simulink model "neural_controller"  (R2017a)
settings: Solver=FixedStepDiscrete  StartTime=0.0  StopTime=inf  FixedStep=0.002  RelTol=1e-3  EnableMultiTasking=on
undefined symbols (not defined in the file or in its folder): HIL
libraries: neural x136, quarc_library x4, simulink x1
(part 3 of 4)

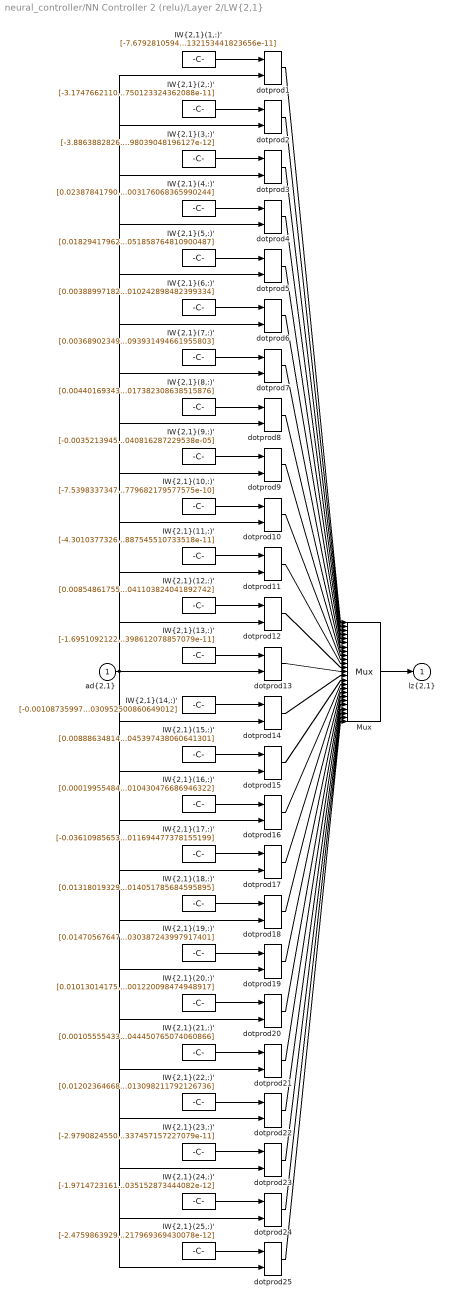
== system neural_controller/NN Controller 2 (relu)/Layer 2/LW{2,1} ==
  "ad{2,1}" : Inport  PortDimensions=25
      mask Display: e = 0.06;c1 = [120 230 180]/255;c2 = ([120 230 180]+0)/(256+128);c3 = ([120 230 180]+128)/(256+128);patch([0 1 1 0],[0 0 1 1],c1);patch([0 1 1 1-e 1-e 0+e],[0 0 1 1-e 0+e 0+e],c2);patch([0 0 1 1-e 0+e 0+e],[0 1 1 1-e 1-e 0+e],c3);plot([0 1 1 0 0],[0 0 1 1 0]);
  "IW{2,1}(1,:)'" : Constant  Value=[-7.6792810594584661e-09;-7.1126316738020698e-11;1.7998320918344641e-08;-2.003723626458679e-10;-1.8516180965883707e-10;-7.5860076472246306e-11;6.2299829523009267e-10;-1.0515209795277028e-10;-1.8827427881449038e-09;2.218470791657716e-11;-3.9406915599531058e-08;1.0151503705757366e-12;-1.9023546382725779e-08;-2.2032313786793295e-10;-2.3151757914767001e-09;-2.9984532169035445e-11;-9.5093536671353531e-12;-5.0992263322406924e-08;-1.3344982605011259e-08;-2.9158255260832613e-09;-1.1630319166261373e-10;-1.2964229482817726e-08;6.1084505465677229e-09;1.0825281524140743e-10;1.8132153441823656e-11]
      mask Display: e = 0.06;c1 = [120 150 230]/255;c2 = ([120 150 230]+0)/383;c3 = ([120 150 230]+128)/383;patch([0 1 1 0],[0 0 1 1],c1);patch([0 1 1 1-e 1-e 0+e],[0 0 1 1-e 0+e 0+e],c2);patch([0 0 1 1-e 0+e 0+e],[0 1 1 1-e 1-e 0+e],c3);plot([0 1 1 0 0],[0 0 1 1 0]);disp('weights');
  "IW{2,1}(10,:)'" : Constant  Value=[-7.539833734705316e-11;-2.4411431451428775e-10;5.9162341033399517e-11;-5.48070123741515e-10;-4.5302392434479749e-10;-2.5669878462677975e-10;1.7387695818048645e-10;-2.2463697075379773e-10;-1.5814520153849316e-10;-1.6547463732050574e-10;-2.9538417906818055e-10;-3.7654524057014066e-12;-2.5148569538890934e-10;-5.7656949292448e-10;2.5000753899474519e-12;-2.4840785547122653e-10;6.2010400842961357e-11;-1.630706221709544e-10;-2.1704856737930736e-10;-8.2373025243356772e-11;-2.9314899085759011e-10;1.8311770093531284e-10;-2.5372084254757587e-10;-4.0386388939167889e-11;-1.2779682179577575e-10]
      mask Display: e = 0.06;c1 = [120 150 230]/255;c2 = ([120 150 230]+0)/383;c3 = ([120 150 230]+128)/383;patch([0 1 1 0],[0 0 1 1],c1);patch([0 1 1 1-e 1-e 0+e],[0 0 1 1-e 0+e 0+e],c2);patch([0 0 1 1-e 0+e 0+e],[0 1 1 1-e 1-e 0+e],c3);plot([0 1 1 0 0],[0 0 1 1 0]);disp('weights');
  "IW{2,1}(11,:)'" : Constant  Value=[-4.301037732631331e-11;-2.569410134808951e-12;-1.0469632599092887e-11;-1.2595773712822758e-12;-1.0156678735682078e-11;-3.4054838340213689e-11;-9.5770075392691075e-12;-1.8306926198411783e-12;-1.0308441497359357e-10;-9.5984236805500613e-11;-1.8259977268230217e-10;-1.9587259074091726e-11;-1.3968105946278729e-10;-1.1647665091168313e-11;-1.3851019848052193e-11;-9.6033937176644037e-12;2.820579720713071e-11;-1.0067866005581733e-10;-1.3484847526334624e-10;-5.6651723409524551e-11;8.5942338897835642e-12;-4.1233821262441008e-12;-1.1667206126410447e-10;-2.6214250577623542e-12;-6.6887545510733518e-11]
      mask Display: e = 0.06;c1 = [120 150 230]/255;c2 = ([120 150 230]+0)/383;c3 = ([120 150 230]+128)/383;patch([0 1 1 0],[0 0 1 1],c1);patch([0 1 1 1-e 1-e 0+e],[0 0 1 1-e 0+e 0+e],c2);patch([0 0 1 1-e 0+e 0+e],[0 1 1 1-e 1-e 0+e],c3);plot([0 1 1 0 0],[0 0 1 1 0]);disp('weights');
  "IW{2,1}(12,:)'" : Constant  Value=[0.0085486175547883157;0.038921469431951253;0.00072928454322535984;-0.005919310881027433;0.0067324029361368288;0.0014729867062613932;0.011651872976152538;0.0096951132432792075;0.014282980967113987;-0.0022472072990480309;0.02697281453022778;0.0033402977445982814;0.066526733165617802;0.0027361323723594641;0.0009416351130375817;0.0060005892677358922;-0.0017547579068491084;0.011895645295689969;0.0058107012873306555;-0.005567481289830826;0.10457499147972557;0.011928304424710184;0.0010842351755472252;0.03450444048361162;0.0041103824041892742]
      mask Display: e = 0.06;c1 = [120 150 230]/255;c2 = ([120 150 230]+0)/383;c3 = ([120 150 230]+128)/383;patch([0 1 1 0],[0 0 1 1],c1);patch([0 1 1 1-e 1-e 0+e],[0 0 1 1-e 0+e 0+e],c2);patch([0 0 1 1-e 0+e 0+e],[0 1 1 1-e 1-e 0+e],c3);plot([0 1 1 0 0],[0 0 1 1 0]);disp('weights');
  "IW{2,1}(13,:)'" : Constant  Value=[-1.6951092122585871e-08;-5.9712221408849155e-11;-4.2727995881829927e-08;-1.5268723788522534e-10;-1.1786285260925152e-10;-6.1318022475459716e-11;-1.4492083639181336e-09;-7.120193341696578e-11;-5.8746453350967224e-09;-1.522926600548734e-11;-7.6277173675718993e-08;5.0409460013806238e-13;-3.5200837251621827e-08;-1.6739184538221271e-10;-5.201417827921483e-09;-7.5605015966112313e-11;7.8486292035284465e-12;-1.0740901393181189e-07;-2.130777853307425e-08;-1.0927906376289981e-09;-7.458065697127481e-11;-5.1051051799692016e-08;-1.3959719228474327e-08;-1.2266524690474954e-11;-1.1398612078857079e-11]
      mask Display: e = 0.06;c1 = [120 150 230]/255;c2 = ([120 150 230]+0)/383;c3 = ([120 150 230]+128)/383;patch([0 1 1 0],[0 0 1 1],c1);patch([0 1 1 1-e 1-e 0+e],[0 0 1 1-e 0+e 0+e],c2);patch([0 0 1 1-e 0+e 0+e],[0 1 1 1-e 1-e 0+e],c3);plot([0 1 1 0 0],[0 0 1 1 0]);disp('weights');
  "IW{2,1}(14,:)'" : Constant  Value=[-0.001087359976365982;0.014994532054224833;-0.00048161962687797658;0.0023381707521366577;0.034947327362041904;0.010589180365643583;0.00037580858668208783;0.0044711535329865354;0.0051232386073423886;-0.00024523223986675933;-0.020647122052367812;0.0037805115068640094;0.12739374876765761;0.030452209012630911;-0.00087797584990192935;0.015370265125823646;-0.038906996003827653;-0.027759582662904993;-0.0086574652701497598;0.013807193556461107;0.062866770256710017;0.008848576139869082;7.7852200123227166e-05;0.066823430685743548;0.0030952500860649012]
      mask Display: e = 0.06;c1 = [120 150 230]/255;c2 = ([120 150 230]+0)/383;c3 = ([120 150 230]+128)/383;patch([0 1 1 0],[0 0 1 1],c1);patch([0 1 1 1-e 1-e 0+e],[0 0 1 1-e 0+e 0+e],c2);patch([0 0 1 1-e 0+e 0+e],[0 1 1 1-e 1-e 0+e],c3);plot([0 1 1 0 0],[0 0 1 1 0]);disp('weights');
  "IW{2,1}(15,:)'" : Constant  Value=[0.0088863481441649201;0.028805562177555567;0.00085740479293599928;-0.010448278624971764;-0.014559925730524618;-0.0052039232464403118;0.010078670622544418;0.0069288194214313942;0.012410948017324149;5.9244647332985789e-05;0.036181882849986205;0.0014764956348752136;0.01593110490784052;-0.017219733564965121;0.001196341715713193;-0.002033634151277173;0.010431016127799078;0.022044008297568363;0.0076614564960669745;-0.018076495184618409;0.0729467409982682;0.010576460114962811;0.0010004496153833981;-0.0063583331762361835;0.0045397438060641301]
      mask Display: e = 0.06;c1 = [120 150 230]/255;c2 = ([120 150 230]+0)/383;c3 = ([120 150 230]+128)/383;patch([0 1 1 0],[0 0 1 1],c1);patch([0 1 1 1-e 1-e 0+e],[0 0 1 1-e 0+e 0+e],c2);patch([0 0 1 1-e 0+e 0+e],[0 1 1 1-e 1-e 0+e],c3);plot([0 1 1 0 0],[0 0 1 1 0]);disp('weights');
  "IW{2,1}(16,:)'" : Constant  Value=[0.00019955484401158415;0.00067388635728634315;1.8997775731461967e-05;-0.0002256414614354404;-0.00027635177889485691;-0.00010088774089898898;0.00023091529890104565;0.00016289364059207442;0.0002845954187697474;1.1933203969252801e-05;0.00079394575255332988;3.7722143976141233e-05;0.00055021284806064342;-0.0003394896127411838;2.6308884670988423e-05;-2.6041962717278154e-05;0.00020427353166977094;0.0004715896170833154;0.00016821614579598878;-0.00037881141697235915;0.0017132367012811396;0.000250579116094033;2.2688109769553548e-05;-5.2576931568082683e-05;0.00010430476686946322]
      mask Display: e = 0.06;c1 = [120 150 230]/255;c2 = ([120 150 230]+0)/383;c3 = ([120 150 230]+128)/383;patch([0 1 1 0],[0 0 1 1],c1);patch([0 1 1 1-e 1-e 0+e],[0 0 1 1-e 0+e 0+e],c2);patch([0 0 1 1-e 0+e 0+e],[0 1 1 1-e 1-e 0+e],c3);plot([0 1 1 0 0],[0 0 1 1 0]);disp('weights');
  "IW{2,1}(17,:)'" : Constant  Value=[-0.036109856536489467;-0.019036186629064276;-0.0054815016316539381;0.06967861303102571;0.061332727846017877;0.0052795114685041198;-0.0051925191815313833;-0.0018808362547497175;-0.0051001745228906395;-0.98650212883476152;-0.29053726241657934;-0.01599267235973249;1.2449192312731583;0.027313731780371622;-0.0091790878449782738;0.0098279050215846452;-0.27375674339103112;-0.27079956763634183;-0.059001072253794591;0.14671588527890911;0.24543718884772109;0.041228611003460536;-0.002497278540755815;1.0645004239809719;-0.00011694477378155199]
      mask Display: e = 0.06;c1 = [120 150 230]/255;c2 = ([120 150 230]+0)/383;c3 = ([120 150 230]+128)/383;patch([0 1 1 0],[0 0 1 1],c1);patch([0 1 1 1-e 1-e 0+e],[0 0 1 1-e 0+e 0+e],c2);patch([0 0 1 1-e 0+e 0+e],[0 1 1 1-e 1-e 0+e],c3);plot([0 1 1 0 0],[0 0 1 1 0]);disp('weights');
  "IW{2,1}(18,:)'" : Constant  Value=[0.013180193294562671;-0.01832335242095794;0.0018687300632919601;-0.026598429671250812;-0.1192523831811606;-0.037681292647196066;0.0046595445016668511;-0.0062180779326500889;0.0050876623668604619;0.0027113534960816889;0.094353915225575083;-0.008205881294492191;-0.29794094749763644;-0.11288884666587964;0.0030523700333772424;-0.043573015575918687;0.083582031303561524;0.085431764893414724;0.020105502131936188;-0.07162657266632845;-0.049990786533464941;-0.0061687796055690811;0.00099094026683705337;-0.21300169631618429;0.0014051785684595895]
      mask Display: e = 0.06;c1 = [120 150 230]/255;c2 = ([120 150 230]+0)/383;c3 = ([120 150 230]+128)/383;patch([0 1 1 0],[0 0 1 1],c1);patch([0 1 1 1-e 1-e 0+e],[0 0 1 1-e 0+e 0+e],c2);patch([0 0 1 1-e 0+e 0+e],[0 1 1 1-e 1-e 0+e],c3);plot([0 1 1 0 0],[0 0 1 1 0]);disp('weights');
  "IW{2,1}(19,:)'" : Constant  Value=[0.014705676471526079;-0.0037914905499059136;0.0019320217527694461;-0.025167320520140802;-0.10492667645076631;-0.033242947282169116;0.0080510037261118644;-0.0024456617849274625;0.0092923766451942381;0.0064911713473241785;0.093334108146343672;-0.006350500228105049;-0.24268427749482493;-0.10005757905756707;0.0030711877779970023;-0.03757539071369137;0.0750431051703635;0.080824464711242633;0.02014862419218081;-0.065499627476395386;-0.01266812952475955;-0.0030906270795722146;0.0012441033357813963;-0.18256389585322375;0.0030387243997917401]
      mask Display: e = 0.06;c1 = [120 150 230]/255;c2 = ([120 150 230]+0)/383;c3 = ([120 150 230]+128)/383;patch([0 1 1 0],[0 0 1 1],c1);patch([0 1 1 1-e 1-e 0+e],[0 0 1 1-e 0+e 0+e],c2);patch([0 0 1 1-e 0+e 0+e],[0 1 1 1-e 1-e 0+e],c3);plot([0 1 1 0 0],[0 0 1 1 0]);disp('weights');
  "IW{2,1}(2,:)'" : Constant  Value=[-3.1747662110966132e-11;7.73937278117594e-12;-3.7463219540287004e-12;-5.9340728255523212e-12;-2.7236647618137786e-12;-4.1883456193740931e-11;7.3694992314728212e-12;-5.3344196383348506e-12;-8.7351651384151508e-11;-7.9982925418328494e-11;-1.4012840818143832e-10;2.8438846222131151e-13;-1.2681316049939503e-10;7.3261463691447547e-13;5.4642931551664244e-12;-1.089076241700762e-11;2.7946339069716205e-11;-9.3284990243965443e-11;-1.11098224269136e-10;-3.736233021564739e-11;-7.9185065671258803e-12;-3.0588242026652366e-12;-8.9017375531224679e-11;-6.9971911726714913e-12;-5.9750123324362088e-11]
      mask Display: e = 0.06;c1 = [120 150 230]/255;c2 = ([120 150 230]+0)/383;c3 = ([120 150 230]+128)/383;patch([0 1 1 0],[0 0 1 1],c1);patch([0 1 1 1-e 1-e 0+e],[0 0 1 1-e 0+e 0+e],c2);patch([0 0 1 1-e 0+e 0+e],[0 1 1 1-e 1-e 0+e],c3);plot([0 1 1 0 0],[0 0 1 1 0]);disp('weights');
  "IW{2,1}(20,:)'" : Constant  Value=[0.01013014175968649;-0.012498606566109946;0.0014217919376139812;-0.020054657772299561;-0.089034158417902326;-0.028145101298815103;0.0038530043220075688;-0.0043517726616277711;0.0042539109661922422;0.0023176727735163783;0.07138270917046452;-0.0060402592245098457;-0.22057473042871267;-0.084368781405189761;0.0023142735131922764;-0.032444695474066011;0.062510062082378234;0.064283472519066437;0.015236329799494694;-0.053744888778392952;-0.034332235462831671;-0.004380518498234549;0.00077480771766379175;-0.15847776405368666;0.001220098474948917]
      mask Display: e = 0.06;c1 = [120 150 230]/255;c2 = ([120 150 230]+0)/383;c3 = ([120 150 230]+128)/383;patch([0 1 1 0],[0 0 1 1],c1);patch([0 1 1 1-e 1-e 0+e],[0 0 1 1-e 0+e 0+e],c2);patch([0 0 1 1-e 0+e 0+e],[0 1 1 1-e 1-e 0+e],c3);plot([0 1 1 0 0],[0 0 1 1 0]);disp('weights');
  "IW{2,1}(21,:)'" : Constant  Value=[0.0010555543300518626;0.0023108869952085005;0.0001140340737172354;-0.00025764674535415014;-0.0020335206928141164;-0.00058363194677767572;0.001015976733930024;0.00052194830220383156;0.0012309537990337566;0.003034245357927848;0.0048571066358807837;-1.8010474050515614e-05;-0.0008171736385963733;-0.0017489116216457131;0.00016742115958282228;-0.00087395919779840981;0.0025258608252747075;0.003543992638676247;0.001082027204315366;-0.001097462565089292;0.0058817508995198005;0.00034873951397666178;0.00011061896876775222;-0.0044380792174932128;0.00044450765074060866]
      mask Display: e = 0.06;c1 = [120 150 230]/255;c2 = ([120 150 230]+0)/383;c3 = ([120 150 230]+128)/383;patch([0 1 1 0],[0 0 1 1],c1);patch([0 1 1 1-e 1-e 0+e],[0 0 1 1-e 0+e 0+e],c2);patch([0 0 1 1-e 0+e 0+e],[0 1 1 1-e 1-e 0+e],c3);plot([0 1 1 0 0],[0 0 1 1 0]);disp('weights');
  "IW{2,1}(22,:)'" : Constant  Value=[0.012023646685503486;-0.016399430115259794;0.0017018603737024665;-0.024187042019239234;-0.10826527256253048;-0.034212024819136842;0.0043048788639688433;-0.0055871994122124952;0.0047097629344176519;0.0025198123677603848;0.08584774552995264;-0.0074326278451825583;-0.27011784762739205;-0.1025051592933013;0.0027781963276783334;-0.039541089455444045;0.075902692834493829;0.077660275130396486;0.01829807684096452;-0.065080988432472217;-0.044788325508654553;-0.0055555191917417736;0.00090661600083301471;-0.19326722570943877;0.0013098211792126736]
      mask Display: e = 0.06;c1 = [120 150 230]/255;c2 = ([120 150 230]+0)/383;c3 = ([120 150 230]+128)/383;patch([0 1 1 0],[0 0 1 1],c1);patch([0 1 1 1-e 1-e 0+e],[0 0 1 1-e 0+e 0+e],c2);patch([0 0 1 1-e 0+e 0+e],[0 1 1 1-e 1-e 0+e],c3);plot([0 1 1 0 0],[0 0 1 1 0]);disp('weights');
  "IW{2,1}(23,:)'" : Constant  Value=[-2.9790824550855467e-11;-6.7120041648906037e-12;-6.0710388600701187e-12;6.8111926946723483e-12;-5.5918771044053318e-12;-5.3716588982021376e-11;7.9204399064392267e-12;-5.5304411013147432e-12;-7.5039652324621861e-11;-1.0979642221447759e-10;-1.8111541917972868e-10;3.6036422567674355e-12;-1.5013353143239249e-10;9.0631795082439541e-12;5.2001717775712573e-12;-8.8846756284766574e-12;5.63369993660505e-11;-8.5663089865284052e-11;-1.4975922319933572e-10;-5.9087910834320275e-11;-1.0976094864108302e-11;-2.2821567234195566e-13;-1.4970013468618046e-10;-3.3131798289421769e-12;-6.2337457157227079e-11]
      mask Display: e = 0.06;c1 = [120 150 230]/255;c2 = ([120 150 230]+0)/383;c3 = ([120 150 230]+128)/383;patch([0 1 1 0],[0 0 1 1],c1);patch([0 1 1 1-e 1-e 0+e],[0 0 1 1-e 0+e 0+e],c2);patch([0 0 1 1-e 0+e 0+e],[0 1 1 1-e 1-e 0+e],c3);plot([0 1 1 0 0],[0 0 1 1 0]);disp('weights');
  "IW{2,1}(24,:)'" : Constant  Value=[-1.9714723161235487e-08;-1.3311802408656901e-11;-4.9745597367239057e-08;-6.1238141909267851e-11;-4.2614013203396124e-11;-2.3751047097339415e-11;-1.745875273838354e-09;-3.1262103553802386e-11;-6.8354121169121968e-09;8.7310823753937401e-12;-8.8780927138340762e-08;8.0689172792817247e-12;-4.0962718389567205e-08;-6.2470140106632016e-11;-6.0661601179792033e-09;-2.5213412563616569e-11;7.8936008881057203e-12;-1.2503704972089463e-07;-2.4798288765834444e-08;-1.2716629166235479e-09;-2.9027139286619137e-11;-5.9460050217482082e-08;-1.62340634639263e-08;-4.9024978961031713e-12;-7.0035152873444082e-12]
      mask Display: e = 0.06;c1 = [120 150 230]/255;c2 = ([120 150 230]+0)/383;c3 = ([120 150 230]+128)/383;patch([0 1 1 0],[0 0 1 1],c1);patch([0 1 1 1-e 1-e 0+e],[0 0 1 1-e 0+e 0+e],c2);patch([0 0 1 1-e 0+e 0+e],[0 1 1 1-e 1-e 0+e],c3);plot([0 1 1 0 0],[0 0 1 1 0]);disp('weights');
  "IW{2,1}(25,:)'" : Constant  Value=[-2.475986392916212e-13;3.5103342751277571e-12;-9.8865432036178798e-13;-3.5781105996286831e-12;1.680453648264645e-12;-9.6435387752281322e-12;1.0839671257044466e-11;-2.3333112413265369e-12;1.6145227362107734e-12;1.0115844357104876e-11;-1.538545584278366e-12;2.9877405143791139e-12;-2.8217741190457491e-12;-3.9461352801403112e-12;-4.4909212344171345e-12;-7.9977565770615599e-12;-1.060594336853036e-11;4.0170778869260341e-12;-1.1289924220125142e-11;-4.8803933824043864e-12;-5.6637584597085797e-12;-1.1211366451726339e-11;-9.5086920530415099e-12;-1.151744751485061e-11;3.7217969369430078e-12]
      mask Display: e = 0.06;c1 = [120 150 230]/255;c2 = ([120 150 230]+0)/383;c3 = ([120 150 230]+128)/383;patch([0 1 1 0],[0 0 1 1],c1);patch([0 1 1 1-e 1-e 0+e],[0 0 1 1-e 0+e 0+e],c2);patch([0 0 1 1-e 0+e 0+e],[0 1 1 1-e 1-e 0+e],c3);plot([0 1 1 0 0],[0 0 1 1 0]);disp('weights');
  "IW{2,1}(3,:)'" : Constant  Value=[-3.8863882826729515e-09;-8.7236645198992326e-12;3.603970721654519e-08;-1.3068868183421996e-12;-8.8122735546962376e-12;-4.6246450436710954e-13;1.0991473834563901e-09;-1.2758449091279944e-11;-4.0923785625092889e-10;9.9829927787223455e-12;-2.3343407056799743e-08;-1.0901018109940021e-11;-1.1834518554835639e-08;-1.3831962085446307e-11;-1.1263358741748662e-09;-2.6282185273417534e-12;6.030387567680668e-12;-2.7312714252359086e-08;-9.4073995884136889e-09;-3.2171861696791232e-09;2.3823661788556188e-12;6.879364424677771e-10;1.205865400955216e-08;1.514331898645933e-11;-9.98039048196127e-12]
      mask Display: e = 0.06;c1 = [120 150 230]/255;c2 = ([120 150 230]+0)/383;c3 = ([120 150 230]+128)/383;patch([0 1 1 0],[0 0 1 1],c1);patch([0 1 1 1-e 1-e 0+e],[0 0 1 1-e 0+e 0+e],c2);patch([0 0 1 1-e 0+e 0+e],[0 1 1 1-e 1-e 0+e],c3);plot([0 1 1 0 0],[0 0 1 1 0]);disp('weights');
  "IW{2,1}(4,:)'" : Constant  Value=[0.023878417904000863;-0.026067123922636486;0.0033203552658731613;-0.046287947654255666;-0.20405883993665144;-0.064518773346212935;0.0096642450015254171;-0.0093423842999586643;0.010764473783257986;0.0063257525323914621;0.16582613371364668;-0.013666627067893646;-0.50147756431859714;-0.19349335838728962;0.0053871303198584474;-0.07422422969371667;0.14364050361718231;0.14857415439413277;0.035450735080039021;-0.12364579065246271;-0.072101489894464063;-0.0095528834486976241;0.0018545884474377983;-0.36234904272976431;0.003176068365990244]
      mask Display: e = 0.06;c1 = [120 150 230]/255;c2 = ([120 150 230]+0)/383;c3 = ([120 150 230]+128)/383;patch([0 1 1 0],[0 0 1 1],c1);patch([0 1 1 1-e 1-e 0+e],[0 0 1 1-e 0+e 0+e],c2);patch([0 0 1 1-e 0+e 0+e],[0 1 1 1-e 1-e 0+e],c3);plot([0 1 1 0 0],[0 0 1 1 0]);disp('weights');
  "IW{2,1}(5,:)'" : Constant  Value=[0.018294179623996869;0.011227153801094326;0.0022556724162024954;-0.025946401053448691;-0.10220234080882376;-0.032391284905276416;0.01273968934703386;0.0012595522230328963;0.015026381503079058;0.013881688658460576;0.10468827992755543;-0.0052101163940022508;-0.21278913839029223;-0.09793632190217999;0.0034987542937795113;-0.036036363277760761;0.075862723378937305;0.086653407459096318;0.022863342307843856;-0.065997212845749081;0.025789102683151439;-0.00021233161333718072;0.0016800993723949957;-0.17418893924732076;0.0051858764810900487]
      mask Display: e = 0.06;c1 = [120 150 230]/255;c2 = ([120 150 230]+0)/383;c3 = ([120 150 230]+128)/383;patch([0 1 1 0],[0 0 1 1],c1);patch([0 1 1 1-e 1-e 0+e],[0 0 1 1-e 0+e 0+e],c2);patch([0 0 1 1-e 0+e 0+e],[0 1 1 1-e 1-e 0+e],c3);plot([0 1 1 0 0],[0 0 1 1 0]);disp('weights');
  "IW{2,1}(6,:)'" : Constant  Value=[0.0038899718296756922;0.0014997290626996673;0.0004877811191189357;-0.0058169338652844021;-0.023307375426379725;-0.0073862479309655211;0.002556843945340398;2.8410045523715898e-05;0.0030025117120920921;0.0026245936018758631;0.022896818043316551;-0.0012573221897862288;-0.050208773603104093;-0.022301520595118723;0.00076177341235290474;-0.0082571690957639089;0.017101460285691508;0.019197998516163363;0.0049831955594062125;-0.014896521352530348;0.0031662079205565402;-0.00024725746915284664;0.00034986576749004058;-0.039974213592965609;0.0010242898482399334]
      mask Display: e = 0.06;c1 = [120 150 230]/255;c2 = ([120 150 230]+0)/383;c3 = ([120 150 230]+128)/383;patch([0 1 1 0],[0 0 1 1],c1);patch([0 1 1 1-e 1-e 0+e],[0 0 1 1-e 0+e 0+e],c2);patch([0 0 1 1-e 0+e 0+e],[0 1 1 1-e 1-e 0+e],c3);plot([0 1 1 0 0],[0 0 1 1 0]);disp('weights');
  "IW{2,1}(7,:)'" : Constant  Value=[0.0036890234955928524;0.0010517852211096401;0.00046631742015422516;-0.0057383355118375053;-0.022898940535637659;-0.0072652453445585909;0.0023630030718752035;-7.3270207869136354e-05;0.0027656577213930767;0.0021238075538849432;0.021976930276934887;-0.001255884541433025;-0.049993713767225542;-0.021934364089302411;0.00073027345004141096;-0.0080960391955342634;0.016637011162296166;0.018532685239488509;0.0047804065568402008;-0.014645717741223236;0.0020224835912702262;-0.00031928030892997418;0.00032875350098849731;-0.039179010455439908;0.00093931494661955803]
      mask Display: e = 0.06;c1 = [120 150 230]/255;c2 = ([120 150 230]+0)/383;c3 = ([120 150 230]+128)/383;patch([0 1 1 0],[0 0 1 1],c1);patch([0 1 1 1-e 1-e 0+e],[0 0 1 1-e 0+e 0+e],c2);patch([0 0 1 1-e 0+e 0+e],[0 1 1 1-e 1-e 0+e],c3);plot([0 1 1 0 0],[0 0 1 1 0]);disp('weights');
  "IW{2,1}(8,:)'" : Constant  Value=[0.0044016934396820737;0.0082973368968054396;0.00048934538021565375;-0.0030467271543566611;-0.012863317393151368;-0.0039616564541080038;0.0040142337759588309;0.0018141595765106449;0.0048373986493036192;0.0085352927149883861;0.021194850860880198;-0.00030495812295295969;-0.01533918216981351;-0.012033035439211458;0.00072700024000165158;-0.0047296399431229841;0.012054812444461384;0.015957336302029612;0.0047118015138530615;-0.0083167893209917364;0.020935406430841918;0.0012257570188019976;0.00045047541805064216;-0.023137944022133365;0.0017382308638515876]
      mask Display: e = 0.06;c1 = [120 150 230]/255;c2 = ([120 150 230]+0)/383;c3 = ([120 150 230]+128)/383;patch([0 1 1 0],[0 0 1 1],c1);patch([0 1 1 1-e 1-e 0+e],[0 0 1 1-e 0+e 0+e],c2);patch([0 0 1 1-e 0+e 0+e],[0 1 1 1-e 1-e 0+e],c3);plot([0 1 1 0 0],[0 0 1 1 0]);disp('weights');
  "IW{2,1}(9,:)'" : Constant  Value=[-0.0035213945118942928;-0.006175563016837915;-0.0005762759115898918;0.0091902001136667261;0.0082520492748213419;0.00093825175724206286;-0.0012405799690018502;-0.0011837729965879732;0.00085928241540028552;-0.11949781573663286;-0.032600682495644524;-0.0023001227650577172;0.1550616503237475;0.0043040612870919037;-0.00097983718150927452;0.0012525551988319455;-0.032800486310620956;-0.030951450017858578;-0.0069495334718673767;0.018973686422027805;0.02757361806087958;0.0038123422326538721;-5.7203904079384138e-05;0.13232435723448521;-6.2040816287229538e-05]
      mask Display: e = 0.06;c1 = [120 150 230]/255;c2 = ([120 150 230]+0)/383;c3 = ([120 150 230]+128)/383;patch([0 1 1 0],[0 0 1 1],c1);patch([0 1 1 1-e 1-e 0+e],[0 0 1 1-e 0+e 0+e],c2);patch([0 0 1 1-e 0+e 0+e],[0 1 1 1-e 1-e 0+e],c3);plot([0 1 1 0 0],[0 0 1 1 0]);disp('weights');
  Mux : Mux  Inputs=25
      mask Display: e = 0.06;c1 = [120 150 230]/255;c2 = ([120 150 230]+0)/383;c3 = ([120 150 230]+128)/383;patch([0 1 1 0],[0 0 1 1],c1);patch([0 1 1 1-e 1-e 0+e],[0 0 1 1-e 0+e 0+e],c2);patch([0 0 1 1-e 0+e 0+e],[0 1 1 1-e 1-e 0+e],c3);plot([0 1 1 0 0],[0 0 1 1 0]);disp('Mux');
  dotprod{1..25} (25 alike) : neural/Weight Functions/dotprod
  "lz{2,1}" : Outport
      mask Display: e = 0.06;c1 = [120 230 180]/255;c2 = ([120 230 180]+0)/(256+128);c3 = ([120 230 180]+128)/(256+128);patch([0 1 1 0],[0 0 1 1],c1);patch([0 1 1 1-e 1-e 0+e],[0 0 1 1-e 0+e 0+e],c2);patch([0 0 1 1-e 0+e 0+e],[0 1 1 1-e 1-e 0+e],c3);plot([0 1 1 0 0],[0 0 1 1 0]);
  wires:
  Mux/1 -> "lz{2,1}"/1
  dotprod25/1 -> Mux/25
  "IW{2,1}(25,:)'"/1 -> dotprod25/1
  dotprod24/1 -> Mux/24
  "IW{2,1}(24,:)'"/1 -> dotprod24/1
  dotprod23/1 -> Mux/23
  "IW{2,1}(23,:)'"/1 -> dotprod23/1
  dotprod22/1 -> Mux/22
  "IW{2,1}(22,:)'"/1 -> dotprod22/1
  dotprod21/1 -> Mux/21
  "IW{2,1}(21,:)'"/1 -> dotprod21/1
  dotprod20/1 -> Mux/20
  "IW{2,1}(20,:)'"/1 -> dotprod20/1
  dotprod19/1 -> Mux/19
  "IW{2,1}(19,:)'"/1 -> dotprod19/1
  dotprod18/1 -> Mux/18
  "IW{2,1}(18,:)'"/1 -> dotprod18/1
  dotprod17/1 -> Mux/17
  "IW{2,1}(17,:)'"/1 -> dotprod17/1
  dotprod16/1 -> Mux/16
  "IW{2,1}(16,:)'"/1 -> dotprod16/1
  dotprod15/1 -> Mux/15
  "IW{2,1}(15,:)'"/1 -> dotprod15/1
  dotprod14/1 -> Mux/14
  "IW{2,1}(14,:)'"/1 -> dotprod14/1
  dotprod13/1 -> Mux/13
  "IW{2,1}(13,:)'"/1 -> dotprod13/1
  dotprod12/1 -> Mux/12
  "IW{2,1}(12,:)'"/1 -> dotprod12/1
  dotprod11/1 -> Mux/11
  "IW{2,1}(11,:)'"/1 -> dotprod11/1
  dotprod10/1 -> Mux/10
  "IW{2,1}(10,:)'"/1 -> dotprod10/1
  dotprod9/1 -> Mux/9
  "IW{2,1}(9,:)'"/1 -> dotprod9/1
  dotprod8/1 -> Mux/8
  "IW{2,1}(8,:)'"/1 -> dotprod8/1
  dotprod7/1 -> Mux/7
  "IW{2,1}(7,:)'"/1 -> dotprod7/1
  dotprod6/1 -> Mux/6
  "IW{2,1}(6,:)'"/1 -> dotprod6/1
  dotprod5/1 -> Mux/5
  "IW{2,1}(5,:)'"/1 -> dotprod5/1
  dotprod4/1 -> Mux/4
  "IW{2,1}(4,:)'"/1 -> dotprod4/1
  dotprod3/1 -> Mux/3
  "IW{2,1}(3,:)'"/1 -> dotprod3/1
  dotprod2/1 -> Mux/2
  "IW{2,1}(2,:)'"/1 -> dotprod2/1
  dotprod1/1 -> Mux/1
  "ad{2,1}"/1 -> dotprod25/2, dotprod24/2, dotprod23/2, dotprod22/2, dotprod21/2, dotprod20/2, dotprod19/2, dotprod18/2, dotprod17/2, dotprod16/2, dotprod15/2, dotprod14/2, dotprod13/2, dotprod12/2, dotprod11/2, dotprod10/2, dotprod9/2, dotprod8/2, dotprod7/2, dotprod6/2, dotprod5/2, dotprod4/2, dotprod3/2, dotprod2/2, dotprod1/2
  "IW{2,1}(1,:)'"/1 -> dotprod1/1

== system neural_controller/NN Controller 2 (relu)/Layer 3/Delays 1 ==
  "p{3}" : Inport  PortDimensions=25
      mask Display: e = 0.06;c1 = [120 230 180]/255;c2 = ([120 230 180]+0)/(256+128);c3 = ([120 230 180]+128)/(256+128);patch([0 1 1 0],[0 0 1 1],c1);patch([0 1 1 1-e 1-e 0+e],[0 0 1 1-e 0+e 0+e],c2);patch([0 0 1 1-e 0+e 0+e],[0 1 1 1-e 1-e 0+e],c3);plot([0 1 1 0 0],[0 0 1 1 0]);
  mux : Mux  Inputs=1
      mask Display: e = 0.06;c1 = [120 150 230]/255;c2 = ([120 150 230]+0)/383;c3 = ([120 150 230]+128)/383;patch([0 1 1 0],[0 0 1 1],c1);patch([0 1 1 1-e 1-e 0+e],[0 0 1 1-e 0+e 0+e],c2);patch([0 0 1 1-e 0+e 0+e],[0 1 1 1-e 1-e 0+e],c3);plot([0 1 1 0 0],[0 0 1 1 0]);disp('Mux')
  "pd{3,2}" : Outport
      mask Display: e = 0.06;c1 = [120 230 180]/255;c2 = ([120 230 180]+0)/(256+128);c3 = ([120 230 180]+128)/(256+128);patch([0 1 1 0],[0 0 1 1],c1);patch([0 1 1 1-e 1-e 0+e],[0 0 1 1-e 0+e 0+e],c2);patch([0 0 1 1-e 0+e 0+e],[0 1 1 1-e 1-e 0+e],c3);plot([0 1 1 0 0],[0 0 1 1 0]);
  wires:
  mux/1 -> "pd{3,2}"/1
  "p{3}"/1 -> mux/1

== system neural_controller/NN Controller 2 (relu)/Layer 3/LW{3,2} ==
  "ad{3,2}" : Inport  PortDimensions=25
      mask Display: e = 0.06;c1 = [120 230 180]/255;c2 = ([120 230 180]+0)/(256+128);c3 = ([120 230 180]+128)/(256+128);patch([0 1 1 0],[0 0 1 1],c1);patch([0 1 1 1-e 1-e 0+e],[0 0 1 1-e 0+e 0+e],c2);patch([0 0 1 1-e 0+e 0+e],[0 1 1 1-e 1-e 0+e],c3);plot([0 1 1 0 0],[0 0 1 1 0]);
  "IW{3,2}(1,:)'" : Constant  Value=[2.5831850497036053e-08;-3.164422580466324e-10;4.8912235148946623e-09;-0.17185495706280574;-0.16871773822086522;-0.034793639541723098;-0.0325536325939981;-0.048290230221108399;0.02603482448541096;-5.1819439166300986e-11;-6.0265520220941646e-10;-0.076950800179635168;1.7871679054175784e-08;0.091321524962058462;-0.10504386376365363;-0.0023999923956929442;0.029568180552103519;-0.090249468444822234;-0.12025722557066551;-0.071218850889115268;-0.012569390168505142;-0.082700043152501207;1.0712734500615271e-10;6.953257971679569e-09;-1.1047697955609369e-12]
      mask Display: e = 0.06;c1 = [120 150 230]/255;c2 = ([120 150 230]+0)/383;c3 = ([120 150 230]+128)/383;patch([0 1 1 0],[0 0 1 1],c1);patch([0 1 1 1-e 1-e 0+e],[0 0 1 1-e 0+e 0+e],c2);patch([0 0 1 1-e 0+e 0+e],[0 1 1 1-e 1-e 0+e],c3);plot([0 1 1 0 0],[0 0 1 1 0]);disp('weights');
  Mux : Mux  Inputs=1
      mask Display: e = 0.06;c1 = [120 150 230]/255;c2 = ([120 150 230]+0)/383;c3 = ([120 150 230]+128)/383;patch([0 1 1 0],[0 0 1 1],c1);patch([0 1 1 1-e 1-e 0+e],[0 0 1 1-e 0+e 0+e],c2);patch([0 0 1 1-e 0+e 0+e],[0 1 1 1-e 1-e 0+e],c3);plot([0 1 1 0 0],[0 0 1 1 0]);disp('Mux');
  dotprod1 : neural/Weight Functions/dotprod
  "lz{3,2}" : Outport
      mask Display: e = 0.06;c1 = [120 230 180]/255;c2 = ([120 230 180]+0)/(256+128);c3 = ([120 230 180]+128)/(256+128);patch([0 1 1 0],[0 0 1 1],c1);patch([0 1 1 1-e 1-e 0+e],[0 0 1 1-e 0+e 0+e],c2);patch([0 0 1 1-e 0+e 0+e],[0 1 1 1-e 1-e 0+e],c3);plot([0 1 1 0 0],[0 0 1 1 0]);
  wires:
  Mux/1 -> "lz{3,2}"/1
  dotprod1/1 -> Mux/1
  "ad{3,2}"/1 -> dotprod1/2
  "IW{3,2}(1,:)'"/1 -> dotprod1/1

== system neural_controller/NN Controller 3 (relu and linear)/Layer 1/Delays 1 ==
  "p{1}" : Inport  PortDimensions=1
      mask Display: e = 0.06;c1 = [120 230 180]/255;c2 = ([120 230 180]+0)/(256+128);c3 = ([120 230 180]+128)/(256+128);patch([0 1 1 0],[0 0 1 1],c1);patch([0 1 1 1-e 1-e 0+e],[0 0 1 1-e 0+e 0+e],c2);patch([0 0 1 1-e 0+e 0+e],[0 1 1 1-e 1-e 0+e],c3);plot([0 1 1 0 0],[0 0 1 1 0]);
  mux : Mux  Inputs=1
      mask Display: e = 0.06;c1 = [120 150 230]/255;c2 = ([120 150 230]+0)/383;c3 = ([120 150 230]+128)/383;patch([0 1 1 0],[0 0 1 1],c1);patch([0 1 1 1-e 1-e 0+e],[0 0 1 1-e 0+e 0+e],c2);patch([0 0 1 1-e 0+e 0+e],[0 1 1 1-e 1-e 0+e],c3);plot([0 1 1 0 0],[0 0 1 1 0]);disp('Mux')
  "pd{1,1}" : Outport
      mask Display: e = 0.06;c1 = [120 230 180]/255;c2 = ([120 230 180]+0)/(256+128);c3 = ([120 230 180]+128)/(256+128);patch([0 1 1 0],[0 0 1 1],c1);patch([0 1 1 1-e 1-e 0+e],[0 0 1 1-e 0+e 0+e],c2);patch([0 0 1 1-e 0+e 0+e],[0 1 1 1-e 1-e 0+e],c3);plot([0 1 1 0 0],[0 0 1 1 0]);
  wires:
  "p{1}"/1 -> mux/1
  mux/1 -> "pd{1,1}"/1

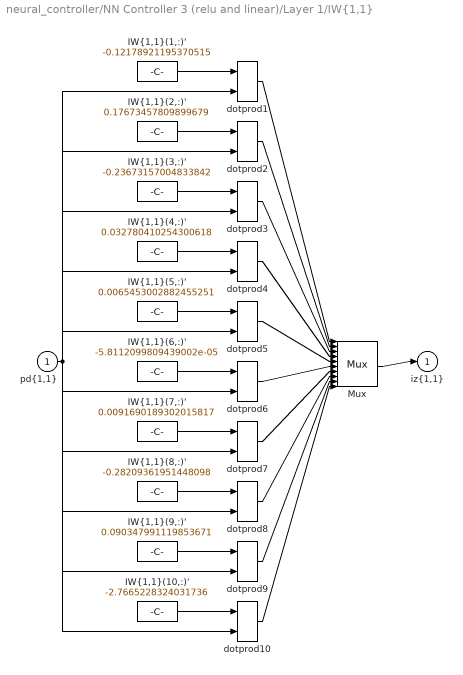
== system neural_controller/NN Controller 3 (relu and linear)/Layer 1/IW{1,1} ==
  "pd{1,1}" : Inport  PortDimensions=1
      mask Display: e = 0.06;c1 = [120 230 180]/255;c2 = ([120 230 180]+0)/(256+128);c3 = ([120 230 180]+128)/(256+128);patch([0 1 1 0],[0 0 1 1],c1);patch([0 1 1 1-e 1-e 0+e],[0 0 1 1-e 0+e 0+e],c2);patch([0 0 1 1-e 0+e 0+e],[0 1 1 1-e 1-e 0+e],c3);plot([0 1 1 0 0],[0 0 1 1 0]);
  "IW{1,1}(1,:)'" : Constant  Value=-0.12178921195370515
      mask Display: e = 0.06;c1 = [120 150 230]/255;c2 = ([120 150 230]+0)/383;c3 = ([120 150 230]+128)/383;patch([0 1 1 0],[0 0 1 1],c1);patch([0 1 1 1-e 1-e 0+e],[0 0 1 1-e 0+e 0+e],c2);patch([0 0 1 1-e 0+e 0+e],[0 1 1 1-e 1-e 0+e],c3);plot([0 1 1 0 0],[0 0 1 1 0]);disp('Weights');
  "IW{1,1}(10,:)'" : Constant  Value=-2.7665228324031736
      mask Display: e = 0.06;c1 = [120 150 230]/255;c2 = ([120 150 230]+0)/383;c3 = ([120 150 230]+128)/383;patch([0 1 1 0],[0 0 1 1],c1);patch([0 1 1 1-e 1-e 0+e],[0 0 1 1-e 0+e 0+e],c2);patch([0 0 1 1-e 0+e 0+e],[0 1 1 1-e 1-e 0+e],c3);plot([0 1 1 0 0],[0 0 1 1 0]);disp('Weights');
  "IW{1,1}(2,:)'" : Constant  Value=0.17673457809899679
      mask Display: e = 0.06;c1 = [120 150 230]/255;c2 = ([120 150 230]+0)/383;c3 = ([120 150 230]+128)/383;patch([0 1 1 0],[0 0 1 1],c1);patch([0 1 1 1-e 1-e 0+e],[0 0 1 1-e 0+e 0+e],c2);patch([0 0 1 1-e 0+e 0+e],[0 1 1 1-e 1-e 0+e],c3);plot([0 1 1 0 0],[0 0 1 1 0]);disp('Weights');
  "IW{1,1}(3,:)'" : Constant  Value=-0.23673157004833842
      mask Display: e = 0.06;c1 = [120 150 230]/255;c2 = ([120 150 230]+0)/383;c3 = ([120 150 230]+128)/383;patch([0 1 1 0],[0 0 1 1],c1);patch([0 1 1 1-e 1-e 0+e],[0 0 1 1-e 0+e 0+e],c2);patch([0 0 1 1-e 0+e 0+e],[0 1 1 1-e 1-e 0+e],c3);plot([0 1 1 0 0],[0 0 1 1 0]);disp('Weights');
  "IW{1,1}(4,:)'" : Constant  Value=0.032780410254300618
      mask Display: e = 0.06;c1 = [120 150 230]/255;c2 = ([120 150 230]+0)/383;c3 = ([120 150 230]+128)/383;patch([0 1 1 0],[0 0 1 1],c1);patch([0 1 1 1-e 1-e 0+e],[0 0 1 1-e 0+e 0+e],c2);patch([0 0 1 1-e 0+e 0+e],[0 1 1 1-e 1-e 0+e],c3);plot([0 1 1 0 0],[0 0 1 1 0]);disp('Weights');
  "IW{1,1}(5,:)'" : Constant  Value=0.0065453002882455251
      mask Display: e = 0.06;c1 = [120 150 230]/255;c2 = ([120 150 230]+0)/383;c3 = ([120 150 230]+128)/383;patch([0 1 1 0],[0 0 1 1],c1);patch([0 1 1 1-e 1-e 0+e],[0 0 1 1-e 0+e 0+e],c2);patch([0 0 1 1-e 0+e 0+e],[0 1 1 1-e 1-e 0+e],c3);plot([0 1 1 0 0],[0 0 1 1 0]);disp('Weights');
  "IW{1,1}(6,:)'" : Constant  Value=-5.8112099809439002e-05
      mask Display: e = 0.06;c1 = [120 150 230]/255;c2 = ([120 150 230]+0)/383;c3 = ([120 150 230]+128)/383;patch([0 1 1 0],[0 0 1 1],c1);patch([0 1 1 1-e 1-e 0+e],[0 0 1 1-e 0+e 0+e],c2);patch([0 0 1 1-e 0+e 0+e],[0 1 1 1-e 1-e 0+e],c3);plot([0 1 1 0 0],[0 0 1 1 0]);disp('Weights');
  "IW{1,1}(7,:)'" : Constant  Value=0.0091690189302015817
      mask Display: e = 0.06;c1 = [120 150 230]/255;c2 = ([120 150 230]+0)/383;c3 = ([120 150 230]+128)/383;patch([0 1 1 0],[0 0 1 1],c1);patch([0 1 1 1-e 1-e 0+e],[0 0 1 1-e 0+e 0+e],c2);patch([0 0 1 1-e 0+e 0+e],[0 1 1 1-e 1-e 0+e],c3);plot([0 1 1 0 0],[0 0 1 1 0]);disp('Weights');
  "IW{1,1}(8,:)'" : Constant  Value=-0.28209361951448098
      mask Display: e = 0.06;c1 = [120 150 230]/255;c2 = ([120 150 230]+0)/383;c3 = ([120 150 230]+128)/383;patch([0 1 1 0],[0 0 1 1],c1);patch([0 1 1 1-e 1-e 0+e],[0 0 1 1-e 0+e 0+e],c2);patch([0 0 1 1-e 0+e 0+e],[0 1 1 1-e 1-e 0+e],c3);plot([0 1 1 0 0],[0 0 1 1 0]);disp('Weights');
  "IW{1,1}(9,:)'" : Constant  Value=0.090347991119853671
      mask Display: e = 0.06;c1 = [120 150 230]/255;c2 = ([120 150 230]+0)/383;c3 = ([120 150 230]+128)/383;patch([0 1 1 0],[0 0 1 1],c1);patch([0 1 1 1-e 1-e 0+e],[0 0 1 1-e 0+e 0+e],c2);patch([0 0 1 1-e 0+e 0+e],[0 1 1 1-e 1-e 0+e],c3);plot([0 1 1 0 0],[0 0 1 1 0]);disp('Weights');
  Mux : Mux  Inputs=10
      mask Display: e = 0.06;c1 = [120 150 230]/255;c2 = ([120 150 230]+0)/383;c3 = ([120 150 230]+128)/383;patch([0 1 1 0],[0 0 1 1],c1);patch([0 1 1 1-e 1-e 0+e],[0 0 1 1-e 0+e 0+e],c2);patch([0 0 1 1-e 0+e 0+e],[0 1 1 1-e 1-e 0+e],c3);plot([0 1 1 0 0],[0 0 1 1 0]);disp('Mux');
  dotprod{1..10} (10 alike) : neural/Weight Functions/dotprod
  "iz{1,1}" : Outport
      mask Display: e = 0.06;c1 = [120 230 180]/255;c2 = ([120 230 180]+0)/(256+128);c3 = ([120 230 180]+128)/(256+128);patch([0 1 1 0],[0 0 1 1],c1);patch([0 1 1 1-e 1-e 0+e],[0 0 1 1-e 0+e 0+e],c2);patch([0 0 1 1-e 0+e 0+e],[0 1 1 1-e 1-e 0+e],c3);plot([0 1 1 0 0],[0 0 1 1 0]);
  wires:
  "IW{1,1}(1,:)'"/1 -> dotprod1/1
  "pd{1,1}"/1 -> dotprod1/2, dotprod2/2, dotprod3/2, dotprod4/2, dotprod5/2, dotprod6/2, dotprod7/2, dotprod8/2, dotprod9/2, dotprod10/2
  dotprod1/1 -> Mux/1
  "IW{1,1}(2,:)'"/1 -> dotprod2/1
  dotprod2/1 -> Mux/2
  "IW{1,1}(3,:)'"/1 -> dotprod3/1
  dotprod3/1 -> Mux/3
  "IW{1,1}(4,:)'"/1 -> dotprod4/1
  dotprod4/1 -> Mux/4
  "IW{1,1}(5,:)'"/1 -> dotprod5/1
  dotprod5/1 -> Mux/5
  "IW{1,1}(6,:)'"/1 -> dotprod6/1
  dotprod6/1 -> Mux/6
  "IW{1,1}(7,:)'"/1 -> dotprod7/1
  dotprod7/1 -> Mux/7
  "IW{1,1}(8,:)'"/1 -> dotprod8/1
  dotprod8/1 -> Mux/8
  "IW{1,1}(9,:)'"/1 -> dotprod9/1
  dotprod9/1 -> Mux/9
  "IW{1,1}(10,:)'"/1 -> dotprod10/1
  dotprod10/1 -> Mux/10
  Mux/1 -> "iz{1,1}"/1

== system neural_controller/NN Controller 3 (relu and linear)/Layer 2/Delays 1 ==
  "p{2}" : Inport  PortDimensions=10
      mask Display: e = 0.06;c1 = [120 230 180]/255;c2 = ([120 230 180]+0)/(256+128);c3 = ([120 230 180]+128)/(256+128);patch([0 1 1 0],[0 0 1 1],c1);patch([0 1 1 1-e 1-e 0+e],[0 0 1 1-e 0+e 0+e],c2);patch([0 0 1 1-e 0+e 0+e],[0 1 1 1-e 1-e 0+e],c3);plot([0 1 1 0 0],[0 0 1 1 0]);
  mux : Mux  Inputs=1
      mask Display: e = 0.06;c1 = [120 150 230]/255;c2 = ([120 150 230]+0)/383;c3 = ([120 150 230]+128)/383;patch([0 1 1 0],[0 0 1 1],c1);patch([0 1 1 1-e 1-e 0+e],[0 0 1 1-e 0+e 0+e],c2);patch([0 0 1 1-e 0+e 0+e],[0 1 1 1-e 1-e 0+e],c3);plot([0 1 1 0 0],[0 0 1 1 0]);disp('Mux')
  "pd{2,1}" : Outport
      mask Display: e = 0.06;c1 = [120 230 180]/255;c2 = ([120 230 180]+0)/(256+128);c3 = ([120 230 180]+128)/(256+128);patch([0 1 1 0],[0 0 1 1],c1);patch([0 1 1 1-e 1-e 0+e],[0 0 1 1-e 0+e 0+e],c2);patch([0 0 1 1-e 0+e 0+e],[0 1 1 1-e 1-e 0+e],c3);plot([0 1 1 0 0],[0 0 1 1 0]);
  wires:
  "p{2}"/1 -> mux/1
  mux/1 -> "pd{2,1}"/1

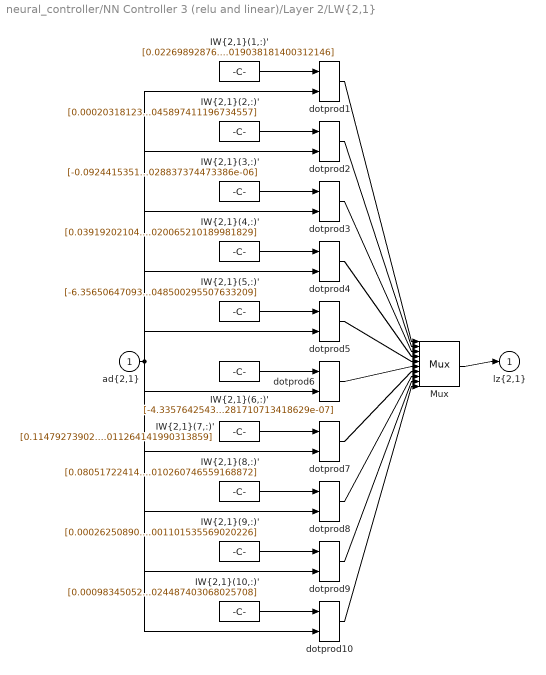
== system neural_controller/NN Controller 3 (relu and linear)/Layer 2/LW{2,1} ==
  "ad{2,1}" : Inport  PortDimensions=10
      mask Display: e = 0.06;c1 = [120 230 180]/255;c2 = ([120 230 180]+0)/(256+128);c3 = ([120 230 180]+128)/(256+128);patch([0 1 1 0],[0 0 1 1],c1);patch([0 1 1 1-e 1-e 0+e],[0 0 1 1-e 0+e 0+e],c2);patch([0 0 1 1-e 0+e 0+e],[0 1 1 1-e 1-e 0+e],c3);plot([0 1 1 0 0],[0 0 1 1 0]);
  "IW{2,1}(1,:)'" : Constant  Value=[0.022698928761215913;-0.094743781100546681;-0.042650657428042429;-0.17725779783636952;0.045879913981159093;-0.042527102843055595;-0.097623224733290548;-0.21048550365863522;-0.029098330323078375;0.019038181400312146]
      mask Display: e = 0.06;c1 = [120 150 230]/255;c2 = ([120 150 230]+0)/383;c3 = ([120 150 230]+128)/383;patch([0 1 1 0],[0 0 1 1],c1);patch([0 1 1 1-e 1-e 0+e],[0 0 1 1-e 0+e 0+e],c2);patch([0 0 1 1-e 0+e 0+e],[0 1 1 1-e 1-e 0+e],c3);plot([0 1 1 0 0],[0 0 1 1 0]);disp('weights');
  "IW{2,1}(10,:)'" : Constant  Value=[0.00098345052625889201;-0.0056338515181384059;0.00012260524211543861;-0.00074922261610023996;0.00075237349334918624;0.00042548678584194874;-0.0047969347519447808;-0.0025460250646606739;-0.0051592342211562517;-0.0024487403068025708]
      mask Display: e = 0.06;c1 = [120 150 230]/255;c2 = ([120 150 230]+0)/383;c3 = ([120 150 230]+128)/383;patch([0 1 1 0],[0 0 1 1],c1);patch([0 1 1 1-e 1-e 0+e],[0 0 1 1-e 0+e 0+e],c2);patch([0 0 1 1-e 0+e 0+e],[0 1 1 1-e 1-e 0+e],c3);plot([0 1 1 0 0],[0 0 1 1 0]);disp('weights');
  "IW{2,1}(2,:)'" : Constant  Value=[0.00020318123110342414;-8.7974402783720868e-06;0.0003493345941487316;-0.00014861398114313583;-4.0459508254219554e-05;-1.8036896512589522e-07;9.8559581055450597e-05;0.00042862695516055789;0.00011813678146352346;0.0045897411196734557]
      mask Display: e = 0.06;c1 = [120 150 230]/255;c2 = ([120 150 230]+0)/383;c3 = ([120 150 230]+128)/383;patch([0 1 1 0],[0 0 1 1],c1);patch([0 1 1 1-e 1-e 0+e],[0 0 1 1-e 0+e 0+e],c2);patch([0 0 1 1-e 0+e 0+e],[0 1 1 1-e 1-e 0+e],c3);plot([0 1 1 0 0],[0 0 1 1 0]);disp('weights');
  "IW{2,1}(3,:)'" : Constant  Value=[-0.092441535163887506;-4.8552451994897163;-0.0011217274193052866;-3.5471710137286516;-0.71899466002773726;-5.0649715365675492e-07;-3.607045008091883;-3.8514795286047865;-1.4638307677886546;-1.2028837374473386e-06]
      mask Display: e = 0.06;c1 = [120 150 230]/255;c2 = ([120 150 230]+0)/383;c3 = ([120 150 230]+128)/383;patch([0 1 1 0],[0 0 1 1],c1);patch([0 1 1 1-e 1-e 0+e],[0 0 1 1-e 0+e 0+e],c2);patch([0 0 1 1-e 0+e 0+e],[0 1 1 1-e 1-e 0+e],c3);plot([0 1 1 0 0],[0 0 1 1 0]);disp('weights');
  "IW{2,1}(4,:)'" : Constant  Value=[0.039192021044091127;0.019473650882432997;0.012852847505145124;-0.2503470259997943;-0.016905756332795938;-0.015666897081268925;0.081469094808243978;-0.11603853386607657;-0.0092466797709826118;-0.020065210189981829]
      mask Display: e = 0.06;c1 = [120 150 230]/255;c2 = ([120 150 230]+0)/383;c3 = ([120 150 230]+128)/383;patch([0 1 1 0],[0 0 1 1],c1);patch([0 1 1 1-e 1-e 0+e],[0 0 1 1-e 0+e 0+e],c2);patch([0 0 1 1-e 0+e 0+e],[0 1 1 1-e 1-e 0+e],c3);plot([0 1 1 0 0],[0 0 1 1 0]);disp('weights');
  "IW{2,1}(5,:)'" : Constant  Value=[-6.3565064709314861e-08;-0.011205985540456296;-0.0083600369624557882;-2.07551839947572e-07;1.2032595311722063e-07;-7.0417632468688732e-08;-0.010870409305483098;-0.0090284579285757564;-0.011272511426957666;-0.0048500295507633209]
      mask Display: e = 0.06;c1 = [120 150 230]/255;c2 = ([120 150 230]+0)/383;c3 = ([120 150 230]+128)/383;patch([0 1 1 0],[0 0 1 1],c1);patch([0 1 1 1-e 1-e 0+e],[0 0 1 1-e 0+e 0+e],c2);patch([0 0 1 1-e 0+e 0+e],[0 1 1 1-e 1-e 0+e],c3);plot([0 1 1 0 0],[0 0 1 1 0]);disp('weights');
  "IW{2,1}(6,:)'" : Constant  Value=[-4.3357642543500272e-06;-4.8343726700954276e-06;3.9234785552437389e-07;-5.2535646026567852e-06;-3.5723495036861346e-06;-3.0005042780489347e-06;-3.8866879214291832e-06;-6.7009962413982064e-06;-1.2266129437397135e-06;3.2281710713418629e-07]
      mask Display: e = 0.06;c1 = [120 150 230]/255;c2 = ([120 150 230]+0)/383;c3 = ([120 150 230]+128)/383;patch([0 1 1 0],[0 0 1 1],c1);patch([0 1 1 1-e 1-e 0+e],[0 0 1 1-e 0+e 0+e],c2);patch([0 0 1 1-e 0+e 0+e],[0 1 1 1-e 1-e 0+e],c3);plot([0 1 1 0 0],[0 0 1 1 0]);disp('weights');
  "IW{2,1}(7,:)'" : Constant  Value=[0.11479273902523091;0.27169735543481482;0.084097849359217353;-0.68435397210225501;-0.11196980164434492;-0.013627873766919794;0.1748750899240108;-0.2790593347865305;0.0088609759777915856;0.011264141990313859]
      mask Display: e = 0.06;c1 = [120 150 230]/255;c2 = ([120 150 230]+0)/383;c3 = ([120 150 230]+128)/383;patch([0 1 1 0],[0 0 1 1],c1);patch([0 1 1 1-e 1-e 0+e],[0 0 1 1-e 0+e 0+e],c2);patch([0 0 1 1-e 0+e 0+e],[0 1 1 1-e 1-e 0+e],c3);plot([0 1 1 0 0],[0 0 1 1 0]);disp('weights');
  "IW{2,1}(8,:)'" : Constant  Value=[0.08051722414811413;-0.48527448633220888;-0.011829325650444013;0.030782806514092903;0.093827683635462955;0.041573179285455349;-0.34554276650886828;-0.096286070570806348;-0.072234635235034553;-0.010260746559168872]
      mask Display: e = 0.06;c1 = [120 150 230]/255;c2 = ([120 150 230]+0)/383;c3 = ([120 150 230]+128)/383;patch([0 1 1 0],[0 0 1 1],c1);patch([0 1 1 1-e 1-e 0+e],[0 0 1 1-e 0+e 0+e],c2);patch([0 0 1 1-e 0+e 0+e],[0 1 1 1-e 1-e 0+e],c3);plot([0 1 1 0 0],[0 0 1 1 0]);disp('weights');
  "IW{2,1}(9,:)'" : Constant  Value=[0.00026250890354311733;-0.0026817979992901832;0.00024513186177763362;-0.0020695903370600227;0.00052970914800821414;-0.00049117690264114701;-0.0021612821810939107;-0.00081764509412338279;-0.0023988544353405581;-0.001101535569020226]
      mask Display: e = 0.06;c1 = [120 150 230]/255;c2 = ([120 150 230]+0)/383;c3 = ([120 150 230]+128)/383;patch([0 1 1 0],[0 0 1 1],c1);patch([0 1 1 1-e 1-e 0+e],[0 0 1 1-e 0+e 0+e],c2);patch([0 0 1 1-e 0+e 0+e],[0 1 1 1-e 1-e 0+e],c3);plot([0 1 1 0 0],[0 0 1 1 0]);disp('weights');
  Mux : Mux  Inputs=10
      mask Display: e = 0.06;c1 = [120 150 230]/255;c2 = ([120 150 230]+0)/383;c3 = ([120 150 230]+128)/383;patch([0 1 1 0],[0 0 1 1],c1);patch([0 1 1 1-e 1-e 0+e],[0 0 1 1-e 0+e 0+e],c2);patch([0 0 1 1-e 0+e 0+e],[0 1 1 1-e 1-e 0+e],c3);plot([0 1 1 0 0],[0 0 1 1 0]);disp('Mux');
  dotprod{1..10} (10 alike) : neural/Weight Functions/dotprod
  "lz{2,1}" : Outport
      mask Display: e = 0.06;c1 = [120 230 180]/255;c2 = ([120 230 180]+0)/(256+128);c3 = ([120 230 180]+128)/(256+128);patch([0 1 1 0],[0 0 1 1],c1);patch([0 1 1 1-e 1-e 0+e],[0 0 1 1-e 0+e 0+e],c2);patch([0 0 1 1-e 0+e 0+e],[0 1 1 1-e 1-e 0+e],c3);plot([0 1 1 0 0],[0 0 1 1 0]);
  wires:
  "IW{2,1}(1,:)'"/1 -> dotprod1/1
  "ad{2,1}"/1 -> dotprod1/2, dotprod2/2, dotprod3/2, dotprod4/2, dotprod5/2, dotprod6/2, dotprod7/2, dotprod8/2, dotprod9/2, dotprod10/2
  dotprod1/1 -> Mux/1
  "IW{2,1}(2,:)'"/1 -> dotprod2/1
  dotprod2/1 -> Mux/2
  "IW{2,1}(3,:)'"/1 -> dotprod3/1
  dotprod3/1 -> Mux/3
  "IW{2,1}(4,:)'"/1 -> dotprod4/1
  dotprod4/1 -> Mux/4
  "IW{2,1}(5,:)'"/1 -> dotprod5/1
  dotprod5/1 -> Mux/5
  "IW{2,1}(6,:)'"/1 -> dotprod6/1
  dotprod6/1 -> Mux/6
  "IW{2,1}(7,:)'"/1 -> dotprod7/1
  dotprod7/1 -> Mux/7
  "IW{2,1}(8,:)'"/1 -> dotprod8/1
  dotprod8/1 -> Mux/8
  "IW{2,1}(9,:)'"/1 -> dotprod9/1
  dotprod9/1 -> Mux/9
  "IW{2,1}(10,:)'"/1 -> dotprod10/1
  dotprod10/1 -> Mux/10
  Mux/1 -> "lz{2,1}"/1

== system neural_controller/NN Controller 3 (relu and linear)/Layer 3/Delays 1 ==
  "p{3}" : Inport  PortDimensions=10
      mask Display: e = 0.06;c1 = [120 230 180]/255;c2 = ([120 230 180]+0)/(256+128);c3 = ([120 230 180]+128)/(256+128);patch([0 1 1 0],[0 0 1 1],c1);patch([0 1 1 1-e 1-e 0+e],[0 0 1 1-e 0+e 0+e],c2);patch([0 0 1 1-e 0+e 0+e],[0 1 1 1-e 1-e 0+e],c3);plot([0 1 1 0 0],[0 0 1 1 0]);
  mux : Mux  Inputs=1
      mask Display: e = 0.06;c1 = [120 150 230]/255;c2 = ([120 150 230]+0)/383;c3 = ([120 150 230]+128)/383;patch([0 1 1 0],[0 0 1 1],c1);patch([0 1 1 1-e 1-e 0+e],[0 0 1 1-e 0+e 0+e],c2);patch([0 0 1 1-e 0+e 0+e],[0 1 1 1-e 1-e 0+e],c3);plot([0 1 1 0 0],[0 0 1 1 0]);disp('Mux')
  "pd{3,2}" : Outport
      mask Display: e = 0.06;c1 = [120 230 180]/255;c2 = ([120 230 180]+0)/(256+128);c3 = ([120 230 180]+128)/(256+128);patch([0 1 1 0],[0 0 1 1],c1);patch([0 1 1 1-e 1-e 0+e],[0 0 1 1-e 0+e 0+e],c2);patch([0 0 1 1-e 0+e 0+e],[0 1 1 1-e 1-e 0+e],c3);plot([0 1 1 0 0],[0 0 1 1 0]);
  wires:
  "p{3}"/1 -> mux/1
  mux/1 -> "pd{3,2}"/1
